simulink model "sim2"  (R2013a)
settings: Solver=ode45  StartTime=0.0  StopTime=4/60  RelTol=1e-3
undefined symbols (not defined in the file): alfa
libraries: powerlib x10, powerlib_extras x2
settings Model: Creator=Guilherme  LastModifiedBy=Guilherme

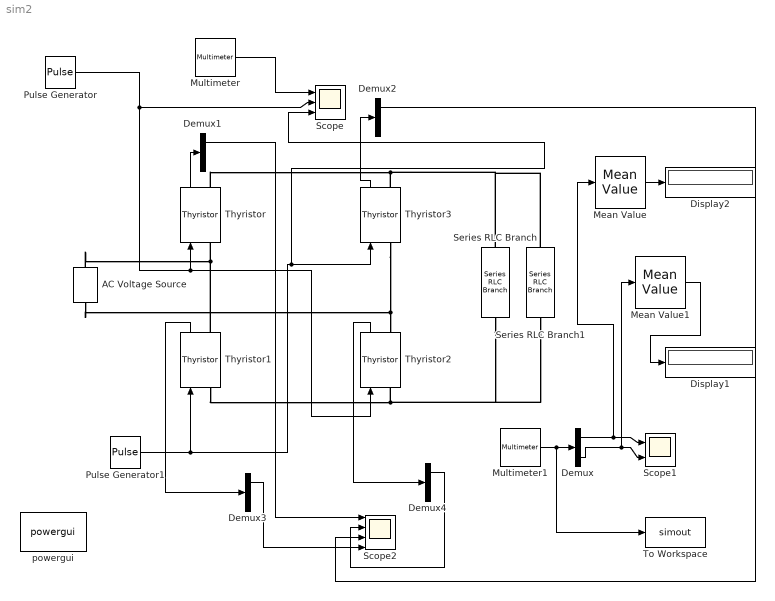
== system sim2 ==
  AC Voltage Source : powerlib/Electrical Sources/AC Voltage Source  Amplitude=100  Phase=0  Frequency=60  SampleTime=0  Measurements=Voltage
  Demux{,1..4} (5 alike) : Demux  Outputs=2
  Display1 : Display
  Display2 : Display
  Mean Value : powerlib_extras/Measurements/Mean Value  Period=1/60
  Mean Value1 : powerlib_extras/Measurements/Mean Value  Period=1/60
  Multimeter : powerlib/Measurements/Multimeter  PhasorSimulation=off  OutputType=Complex  sel=3  L=5  Gain=1  yselected={'Usrc: AC Voltage Source'};  PSBOutputType=1  PSBequivalent=0  AxesSetting=[0,0.1,-100,100]  Display=0  SavedBlockNames=-11
  Multimeter1 : powerlib/Measurements/Multimeter  PhasorSimulation=off  OutputType=Complex  sel=[1 4]  L=5  Gain=[1 1]  yselected={'Ub: Series RLC Branch','Ib: Series RLC Branch'};  PSBOutputType=1  PSBequivalent=0  AxesSetting=[0,0.1,-100,100]  Display=0  SavedBlockNames=-11
  Pulse Generator : DiscretePulseGenerator  PulseType=Time based  Period=1/60  PhaseDelay=alfa/360/60
  Pulse Generator1 : DiscretePulseGenerator  PulseType=Time based  Period=1/60  PhaseDelay=(alfa+180)/360/60
  Scope : Scope  NumInputPorts=3
      settings: YMin=-5~-5~-5  YMax=5~5~5
  Scope1 : Scope  NumInputPorts=2
      settings: YMin=-5~-5  YMax=5~5
  Scope2 : Scope  NumInputPorts=4
      settings: YMin=-5~-5~-5~-5  YMax=5~5~5~5  SaveName=ScopeData2
  Series RLC Branch : powerlib/Elements/Series RLC Branch  LConnTagsString=__new0  RConnTagsString=__new0  BranchType=R  Resistance=50  Inductance=100e-3  SetiL0=off  InitialCurrent=0  Capacitance=1e-6  Setx0=off  InitialVoltage=0  Measurements=Branch voltage and current
  Series RLC Branch1 : powerlib/Elements/Series RLC Branch  LConnTagsString=__new0  RConnTagsString=__new0  BranchType=C  Resistance=50  Inductance=100e-3  SetiL0=off  InitialCurrent=0  Capacitance=1e-3  Setx0=off  InitialVoltage=0  Measurements=Branch voltage and current
  Thyristor{,1..3} (4 alike) : powerlib/Power Electronics/Thyristor  Ron=0.001  Lon=0  Vf=0.8  IC=0  Rs=500  Cs=250e-9  Measurements=on
  To Workspace : ToWorkspace  VariableName=simout  SampleTime=-1  SaveFormat=Timeseries
  powergui : powerlib/powergui  Priority=1  SimulationMode=Continuous  SolverType=Tustin  SampleTime=50e-6  frequency=60  SPID=off  DisableSnubberDevices=off  DisableRonSwitches=off  DisableVfSwitches=off  SwTol=0  Interpol=off  DisplayEquations=off  frequencyindice=60  Pbase=100e6  ErrMax=1e-4  Iterations=50  UnitsV=kV  UnitsW=MW  FunctionMessages=off  echomessages=off  HookPort=off  EnableUseOfTLC=off  x0status=blocks  RestoreLinks=warning  ResistiveCurrentMeasurement=off  Frange=[0:2:500]  Ylog=off  Xlog=on  ShowGrid=off  save=off  variable=ZData  ZoomFFT=off  StartTime=0.0  cycles=1  DisplayStyle=1  fundamental=60  FreqAxis=off  MaxFrequency=1000  frequencyindicesteady=1  RmsSteady=1  display=off  Ts=0  methode=off
  wires:
  Pulse Generator/1 -> Thyristor2/1, Thyristor/1, Scope/2
  Pulse Generator1/1 -> Scope/3, Thyristor3/1, Thyristor1/1
  Multimeter/1 -> Scope/1
  Multimeter1/1 -> To Workspace/1, Demux/1
  Demux/2 -> Mean Value1/1, Scope1/2
  Demux/1 -> Mean Value/1, Scope1/1
  Thyristor/1 -> Demux1/1
  Thyristor3/1 -> Demux2/1
  Thyristor1/1 -> Demux3/1
  Thyristor2/1 -> Demux4/1
  Demux1/1 -> Scope2/1
  Demux4/1 -> Scope2/2
  Demux2/1 -> Scope2/3
  Demux3/1 -> Scope2/4
  Mean Value/1 -> Display2/1
  Mean Value1/1 -> Display1/1
  connections:
  Thyristor1/RConn1 -- AC Voltage Source/RConn1 -- Thyristor/LConn1
  Thyristor3/LConn1 -- AC Voltage Source/LConn1 -- Thyristor2/RConn1
  Thyristor3/RConn1 -- Series RLC Branch1/LConn1 -- Series RLC Branch/LConn1 -- Thyristor/RConn1
  Thyristor1/LConn1 -- Series RLC Branch1/RConn1 -- Series RLC Branch/RConn1 -- Thyristor2/LConn1
